simulink model "dynamics_with_control"  (R2023b)
settings: Solver=ode45  StartTime=0.0  StopTime=StopTime  FixedStep=.1  RelTol=1e-5
PreLoadFcn:
  | gravity = true;
  | e_a = 504;
  | e_b = 496;
  | k = 10;
  | b = 10;
  | ktr = 10;
  | btr = 10;
  | ks = 0.1;
  | bs = 10;
  | d0 = 125;
  | l0 = 615.3882;
  | p0 = 100;
  | ls0 = 707.1068;
  | w = -0.007;
  | kp_M = 0.1;
  | ki_M = 0.0023;
  | mu = 398600000000000;
  | mp = 1500;
  | mp_inv = 0.00066667;
  | mtr = 1.6667;
  | mtr_inv = 0.6;
  | NRao0 = [499.999999999579;-4.21217266566732e-10;6878000];
  | NRbo0 = [-500.000000000421;-4.21094801886817e-10;6878000];
  | NRfo0 = [-4.21186650396753e-10;-4.21186650396753e-10;6878500];
  | NRgo0 = [-4.21125418056796e-10;-4.21125418056796e-10;6877500];
  | NRdo0 = [-4.21171342311764e-10;-125.000000000421;6878000];
  | NReo0 = [-4.21140726141785e-10;124.999999999579;6878000];
  | NVao0 = [7612.67977015526;-9.32070078155593e-13;-3.49999999999953];
  | NVbo0 = [7612.67977015526;-9.32498704535295e-13;3.50000000000047];
  | NVfo0 = [7616.17977015526;-9.32713017725146e-13;4.66356508862573e-13];
  | NVgo0 = [7609.17977015526;-9.31855764965743e-13;4.65927882482871e-13];
  | NVdo0 = [7612.67977015526;-9.32284391345444e-13;4.66142195672722e-13];
  | NVeo0 = [7612.67977015526;-9.32284391345444e-13;4.66142195672722e-13];
PostLoadFcn:
  | StopTime = 3000;
values from neighbouring files (symbols this model uses):
  truss_length = 250    [main.m]
libraries: matrix_library x16, vrlib x14
(part 2 of 2)

== matlab function dynamics_with_control/Tether Length Controller/MATLAB Function2 ==
  data: lref output; q input; a input; b input; half_tr input
function lref = q2ref(q,a,b,half_tr)
psi = pi/4;
if q(3) < 0
    q4 = -q(4);
else
    q4 = q(4);
end
phi = 2 * acos(q4);
r = sqrt(a^2 * b^2 / (b^2*cos(phi+psi)^2 + a^2*sin(phi+psi)^2));
lref = sqrt(r^2 + half_tr^2);

== matlab function dynamics_with_control/Tether Length Controller/MATLAB Function1 ==
  data: lref output; q input; a input; b input; half_tr input
function lref = q2ref(q,a,b,half_tr)
psi = pi/4;
if q(3) < 0
    q4 = -q(4);
else
    q4 = q(4);
end
phi = 2 * acos(q4);
r = sqrt(a^2 * b^2 / (b^2*cos(phi+psi)^2 + a^2*sin(phi+psi)^2));
lref = sqrt(r^2 + half_tr^2);

== matlab function dynamics_with_control/Anguar Momentum Controller/pinv1 ==
  data: u input; y output
function y = fcn(u)

y = pinv(u);
